simulink model "task_3"  (R2023a)
settings: Solver=VariableStepAuto  StartTime=0.0  StopTime=10.0  RelTol=1e-8
settings Model: Creator=user  LastModifiedBy=user

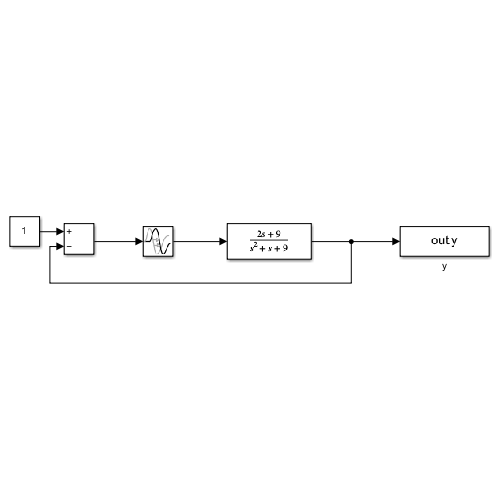
[thumbnail: Simulink's stored preview of the top-level diagram]
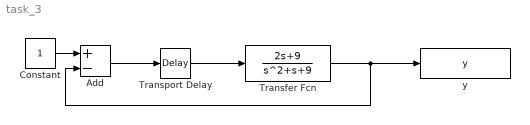
== system task_3 ==
  Add : Sum  Inputs=+-
  Constant : Constant  SampleTime=-1
  Transfer Fcn : TransferFcn  Numerator=[2, 9]  Denominator=[1, 1, 9]
  Transport Delay : TransportDelay  DelayTime=0.5  BufferSize=3072
  y : ToWorkspace  VariableName=y  SaveFormat=Timeseries  SampleTime=-1
  wires:
  Transport Delay/1 -> Transfer Fcn/1
  Add/1 -> Transport Delay/1
  Constant/1 -> Add/1
  Transfer Fcn/1 -> Add/2, y/1
